simulink model "Paper_Simulation_final"  (R2020a)
settings: Solver=ode15s  StartTime=0.0  StopTime=1  MaxStep=0.000002  MinStep=2e-12  RelTol=1e-3
model workspace (MAT data in the model file):
  Wo = 1
  wfinal = Simulink.Parameter
  wfinal.DataType = 'auto'
  wfinal.Dimensions = [0 0]
values from neighbouring files (symbols this model uses):
  a = sqrt(2)*sigma    [tune.m]
  A = conv(A,[1 .5 1])    [tune.m]
  ades = 2*zeta    [tune.m]
  B = conv(B,[-1.5 1])    [tune.m]
  beta = beta/fact    (= 0.5)    [tune.m]
  d = [0*(1:Td/h) 1]    [tune.m]
  d1 = [0*(1:round(Tdhat/h)) 1]    [tune.m]
  h = Tmax/Npts    [tune.m]
  K = K/fact    [tune.m]
  K0 = 1/Kp0    [tune.m]
  K_hat = TThat*ppp(2)/stepsize    [tune.m]
  kfinal = 1/Kw    [tune.m]
  Kmult = 1*Kmult    [tune.m]
  load_s = -0.000    (= 0)    [tune.m]
  phi_c = -1.25; end    [tune.m]
  SetPoint = 1    [tune.m]
  Sn = Snset*st    (= 0)    [tune.m]
  st = 0.1    [tune.m]
  stepsize = 1/Tmax    [tune.m]
  T_l = 0    [tune.m]
  Td = max(h*round(Td/h),h)    [tune.m]
  Tf = Tf*fact    [tune.m]
  Tmax = Tmax_n    [tune.m]
  Tmax_c = Tmax_c+T_l    [tune.m]
  Ts = max((2*Tmhat-Tdhat),ty2)    [tune.m]
  Tsw = max(10*Tmhat,5/(beta*wbar))    [tune.m]
  TswK = Tsw/2    [tune.m]
  TThat = -0.5*ppp(2)/ppp(1)    [tune.m]
  wbar = wbar_n    [tune.m]
  wfinal = wbar_n    [tune.m]
undefined symbols (not defined in the file or in its folder): fdesignblkfcn, gcbh, tstop
libraries: simulink x3, simulink_extras x3, powerlib_meascontrol x2
settings Model: Creator=Ayush Agrawal  LastModifiedBy=Ayush Agrawal
settings SolverCC: InitialStep=2e-6  ZeroCrossAlgorithm=Adaptive
settings DebuggingCC: AlgebraicLoopMsg=none

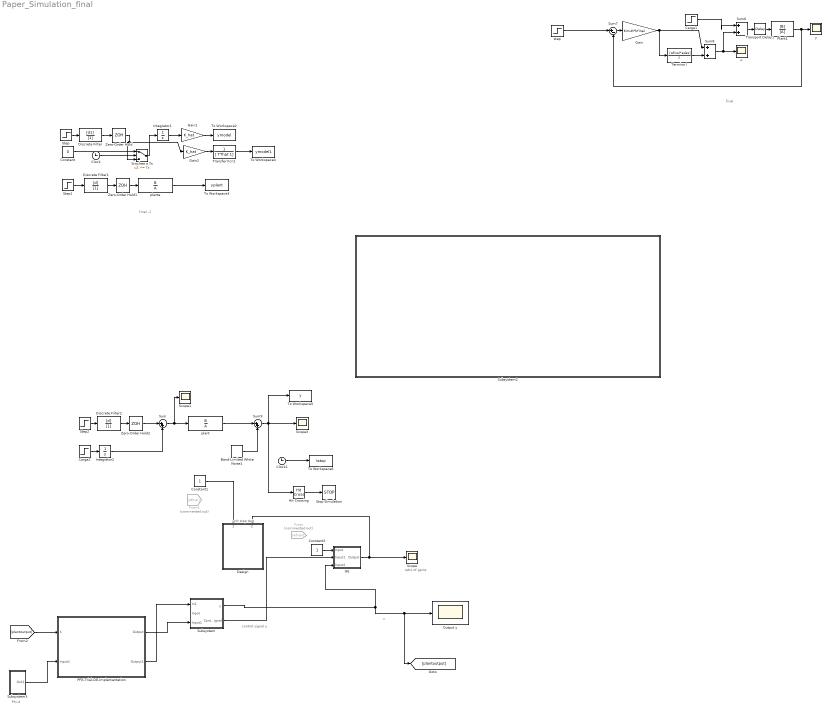
== system Paper_Simulation_final ==
  note: ratio of gains
  note: x
  note: Phi-d
  note: control signal
      |         u
  note: final -1
  note: final
  note: unit step test
  Band-Limited White Noise1 : simulink/Sources/Band-Limited White Noise  Cov=[Sn]  Ts=h  seed=[23341]
  Carga1 : Step  Time=0  After=load  SampleTime=0
  Carga2 : Step  Time=T_l  After=load_s  SampleTime=0
  Clock : Clock
  Clock1 : Clock
  Constant : Constant  Value=0
  Constant1 : Constant
  Constant2 : Constant
  Design : Subsystem  mask{a=1.5}
  Discrete Filter : DiscreteFilter  Numerator=[d1]  Denominator=[1]  SampleTime=h
  Discrete Filter1 : DiscreteFilter  Numerator=[d]  Denominator=[1]  SampleTime=h
  Discrete Filter2 : DiscreteFilter  Numerator=[d]  Denominator=[1]  SampleTime=h
  From : From  Commented=on  GotoTag=wfinal
  From1 : From  Commented=on  GotoTag=wfinal
  GE : Subsystem  mask{winitial=10}
  Gain : Gain  Gain=Kmult*kfinal  SaturateOnIntegerOverflow=on  OutDataTypeStr=Inherit: Same as input  ParamDataTypeStr=Inherit: Same as input
  Gain1 : Gain  Gain=K_hat  SaturateOnIntegerOverflow=on  OutDataTypeStr=Inherit: Same as input  ParamDataTypeStr=Inherit: Same as input
  Gain2 : Gain  Gain=K_hat  SaturateOnIntegerOverflow=on  OutDataTypeStr=Inherit: Same as input  ParamDataTypeStr=Inherit: Same as input
  Hit Crossing : HitCross  HitCrossingOffset=Y2  HitCrossingDirection=rising
  Integrator1 : Integrator
  Integrator2 : Integrator
  Output y : Scope
  PFE-Trial-DE-Implementation : Subsystem  mask{winitial=10}
  Plant1 : TransferFcn  Numerator=[B]  Denominator=[A]
  Scope : Scope
  Scope1 : Scope
  Scope3 : Scope
  Siwchea a Ts : Switch  Threshold=Ts  SaturateOnIntegerOverflow=on
  Step : Step  Time=0  After=stepsize  SampleTime=h
  Step1 : Step  Time=0  After=stepsize  SampleTime=h
  Step2 : Step  Time=0  After=stepsize  SampleTime=h
  Stop Simulation : Stop
  Subsystem : Subsystem  mask{Ti=1, r=0.25}
  Subsystem2 : Subsystem
  Subsystem3 : Subsystem  mask{Phid=10}
      mask prompts: Phid "Phi-d"
  Sum{,6,8..9} (4 alike) : Sum  Inputs=|++  InputSameDT=on  SaturateOnIntegerOverflow=on  OutDataTypeStr=Inherit: Same as first input
  Sum7 : Sum  Inputs=|+-  InputSameDT=on  SaturateOnIntegerOverflow=on  OutDataTypeStr=Inherit: Same as first input
  Termino I : TransferFcn  Numerator=[wfinal*ades]  Denominator=[1 0]
  To Workspace2 : ToWorkspace  VariableName=ymodel  SampleTime=h
  To Workspace3 : ToWorkspace  VariableName=yplant  SampleTime=h
  To Workspace4 : ToWorkspace  VariableName=ymodel1  SampleTime=h
  To Workspace5 : ToWorkspace  VariableName=y  SampleTime=h
  To Workspace6 : ToWorkspace  VariableName=tstop  SampleTime=h
      settings: MaxDataPoints=1
  Transfer Fcn1 : TransferFcn  Denominator=[ TThat 1]
  Transport Delay1 : TransportDelay  DelayTime=Td  BufferSize=16384
  Zero-Order Hold : ZeroOrderHold  SampleTime=h
  Zero-Order Hold1 : ZeroOrderHold  SampleTime=h
  Zero-Order Hold2 : ZeroOrderHold  SampleTime=h
  plant : TransferFcn  Numerator=B  Denominator=A
  planta : TransferFcn  Numerator=B  Denominator=A
  step : Step  Time=0  After=SetPoint  SampleTime=0
  u : Scope
  y : Scope
  wires:
  Subsystem/1(y) -> GE/3(Input2), [plantoutput], Output y/1
  GE/1(Output) -> Scope/1, Design/2(Plant Gain Amplitude)
  Subsystem3/1(Out1) -> PFE-Trial-DE-Implementation/2(Input1)
  [plantoutput] -> PFE-Trial-DE-Implementation/1(X)
  Subsystem/2(Control SIgnal) -> GE/2(Input1)
  Constant1/1 -> Design/1(PFE O/P frequency)
  Constant2/1 -> GE/1(Input)
  PFE-Trial-DE-Implementation/1(Output) -> Subsystem/3(Input1)
  PFE-Trial-DE-Implementation/2(Output1) -> Subsystem/1(In1)
  Transfer Fcn1/1 -> To Workspace4/1
  Discrete Filter1/1 -> Zero-Order Hold1/1
  Gain2/1 -> Transfer Fcn1/1
  Integrator1/1 -> Gain1/1
  Step1/1 -> Discrete Filter1/1
  Siwchea a Ts/1 -> Integrator1/1
  Constant/1 -> Siwchea a Ts/1
  Step/1 -> Discrete Filter/1
  Discrete Filter/1 -> Zero-Order Hold/1
  Zero-Order Hold/1 -> Siwchea a Ts/3, Gain2/1
  planta/1 -> To Workspace3/1
  Gain1/1 -> To Workspace2/1
  Clock/1 -> Siwchea a Ts/2
  Zero-Order Hold1/1 -> planta/1
  Plant1/1 -> Sum7/2, y/1
  Sum7/1 -> Gain/1
  Sum8/1 -> Sum6/2, u/1
  Carga1/1 -> Sum6/1
  step/1 -> Sum7/1
  Gain/1 -> Sum8/1, Termino I/1
  Termino I/1 -> Sum8/2
  Transport Delay1/1 -> Plant1/1
  Sum6/1 -> Transport Delay1/1
  Discrete Filter2/1 -> Zero-Order Hold2/1
  Carga2/1 -> Integrator2/1
  Step2/1 -> Discrete Filter2/1
  Hit Crossing/1 -> Stop Simulation/1
  Band-Limited White Noise1/1 -> Sum9/2
  Zero-Order Hold2/1 -> Sum/1
  Integrator2/1 -> Sum/2
  Clock1/1 -> To Workspace6/1
  Sum9/1 -> Scope3/1, To Workspace5/1, Hit Crossing/1
  plant/1 -> Sum9/1
  Sum/1 -> plant/1, Scope1/1

== system Paper_Simulation_final/Design ==
  PFE O/P frequency : Inport
  Plant Gain Amplitude : Inport  Port=2
  Goto1 : Goto  Commented=on  GotoTag=Ti  TagVisibility=global
  Scope : Scope
  Scope1 : Scope
  Subsystem : Subsystem
  tag scope: K=global
  wires:
  PFE O/P frequency/1 -> Subsystem/1(PFE O/P freq)
  Plant Gain Amplitude/1 -> Subsystem/2(Input)
  Subsystem/1(K) -> Scope/1, [K]
  Subsystem/2(Ti) -> Scope1/1, Goto1/1

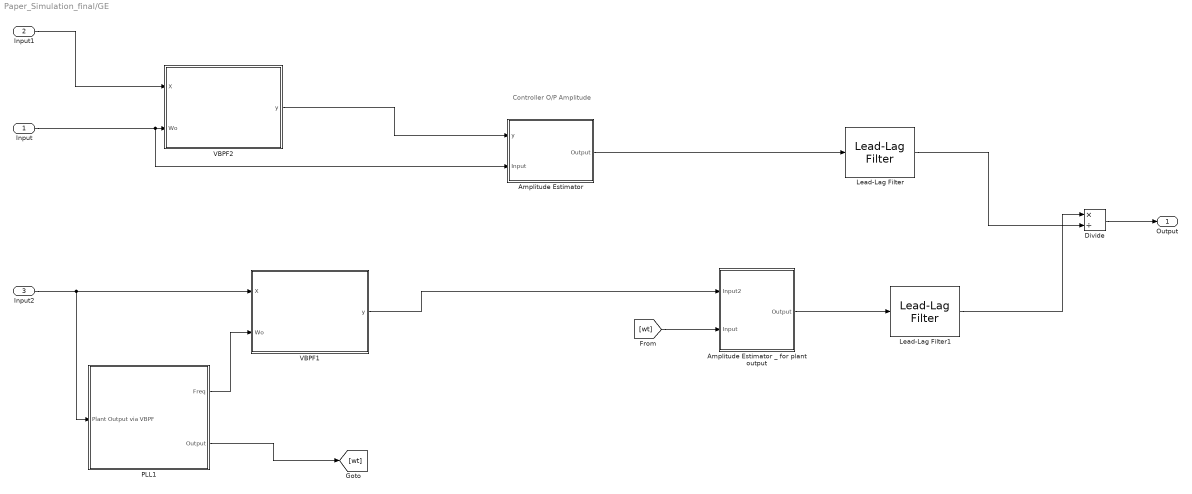
== system Paper_Simulation_final/GE ==
  note: Controller O/P Amplitude
  Input : Inport
  Input1 : Inport  Port=2
  Input2 : Inport  Port=3
  Amplitude Estimator : Subsystem
  Amplitude Estimator _ for plant output : Subsystem
  Divide : Product  Inputs=*/
  Lead-Lag Filter : powerlib_meascontrol/Filters/Lead-Lag Filter  T1=0  T2=10/winitial  Vdc_Init=0  Ts=0.1
      settings: SourceProductBaseCode=PS
  Lead-Lag Filter1 : powerlib_meascontrol/Filters/Lead-Lag Filter  T1=0  T2=10/winitial  Vdc_Init=0  Ts=0
      settings: SourceProductBaseCode=PS
  PLL1 : Subsystem
  VBPF1 : Subsystem
  VBPF2 : Subsystem
  Output : Outport
  wires:
  Input1/1 -> VBPF2/1(X)
  Input2/1 -> PLL1/1(Plant Output via VBPF), VBPF1/1(X)
  Amplitude Estimator _ for plant output/1(Output) -> Lead-Lag Filter1/1
  Divide/1 -> Output/1
  Lead-Lag Filter1/1 -> Divide/1
  Lead-Lag Filter/1 -> Divide/2
  PLL1/1(Freq) -> VBPF1/2(Wo)
  PLL1/2(Output) -> [wt]
  Input/1 -> Amplitude Estimator/2(Input), VBPF2/2(Wo)
  VBPF1/1(y) -> Amplitude Estimator _ for plant output/1(Input2)
  VBPF2/1(y) -> Amplitude Estimator/1(y)
  [wt] -> Amplitude Estimator _ for plant output/2(Input)
  Amplitude Estimator/1(Output) -> Lead-Lag Filter/1

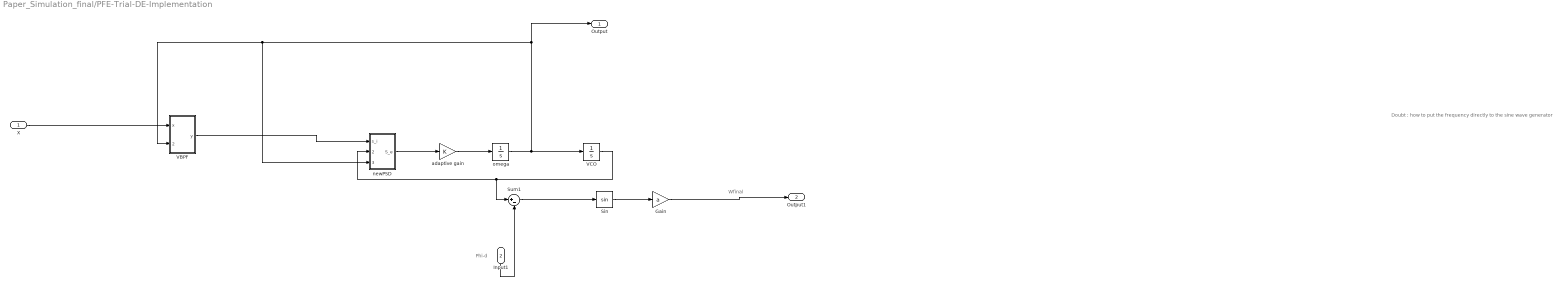
== system Paper_Simulation_final/PFE-Trial-DE-Implementation ==
  note: Doubt : how to put the frequency directly to the sine wave generator
  note: Wfinal
  note: Phi-d
  X : Inport
  Input1 : Inport  Port=2
  "   adaptive gain" : Gain  Gain=K  SaturateOnIntegerOverflow=on  OutDataTypeStr=Inherit: Same as input  ParamDataTypeStr=Inherit: Same as input
  Gain : Gain  Gain=a
  Sin : Trigonometry
  Sum1 : Sum  Inputs=|+-
  VBPF : Subsystem
  "VCO " : Integrator  InitialCondition=-pi  LowerSaturationLimit=0.5
  newPSD : Subsystem
  omega : Integrator  InitialCondition=wbar  LowerSaturationLimit=wbar/3
  Output : Outport
  Output1 : Outport  Port=2
  wires:
  Input1/1 -> Sum1/2
  X/1 -> VBPF/1(x)
  Sum1/1 -> Sin/1
  Sin/1 -> Gain/1
  Gain/1 -> Output1/1
  ? -> ?
  VBPF/1(y) -> newPSD/1(s_i)
  newPSD/1(S_e) -> "   adaptive gain"/1
  "   adaptive gain"/1 -> omega/1
  omega/1 -> Output/1, VBPF/2(omega_0), newPSD/3(omega_o), "VCO "/1
  "VCO "/1 -> newPSD/2(phi_o), Sum1/1

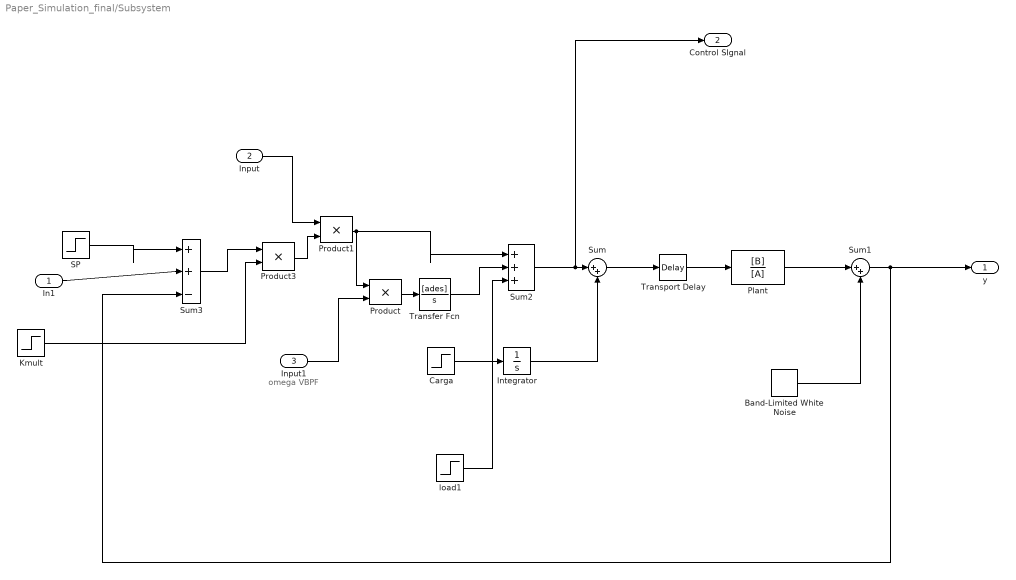
== system Paper_Simulation_final/Subsystem ==
  note: omega VBPF
  In1 : Inport
  Input : Inport  Port=2
  Input1 : Inport  Port=3
  Band-Limited White Noise : simulink/Sources/Band-Limited White Noise  Cov=[Sn]  Ts=st  seed=[23341]
  Carga : Step  Time=T_l  After=load_s  SampleTime=0
  Integrator : Integrator
  Kmult : Step  Time=tstop  After=Kmult  SampleTime=0
  Plant : TransferFcn  Numerator=[B]  Denominator=[A]
  Product : Product  InputSameDT=on  SaturateOnIntegerOverflow=on  OutDataTypeStr=Inherit: Same as first input
  Product1 : Product  InputSameDT=on  SaturateOnIntegerOverflow=on  OutDataTypeStr=Inherit: Same as first input
  Product3 : Product  InputSameDT=on  SaturateOnIntegerOverflow=on  OutDataTypeStr=Inherit: Same as first input
  SP : Step  Time=Tmax_c/2  Before=SetPoint  After=SetPoint  SampleTime=0
  Sum : Sum  Inputs=|++
  Sum1 : Sum  Inputs=|++  InputSameDT=on  SaturateOnIntegerOverflow=on  OutDataTypeStr=Inherit: Same as first input
  Sum2 : Sum  Inputs=|+++
  Sum3 : Sum  Inputs=|++-  InputSameDT=on  SaturateOnIntegerOverflow=on  OutDataTypeStr=Inherit: Same as first input
  Transfer Fcn : TransferFcn  Numerator=[ades]  Denominator=[1 0]
  Transport Delay : TransportDelay  DelayTime=Td  BufferSize=65536
  load1 : Step  Time=Tmax  Before=stepsize  After=stepsize  SampleTime=0
  y : Outport
  Control SIgnal : Outport  Port=2
  wires:
  Plant/1 -> Sum1/1
  Band-Limited White Noise/1 -> Sum1/2
  Transport Delay/1 -> Plant/1
  Sum/1 -> Transport Delay/1
  Carga/1 -> Integrator/1
  Integrator/1 -> Sum/2
  Sum2/1 -> Control SIgnal/1, Sum/1
  Transfer Fcn/1 -> Sum2/2
  load1/1 -> Sum2/3
  In1/1 -> Sum3/2
  SP/1 -> Sum3/1
  Sum3/1 -> Product3/1
  Kmult/1 -> Product3/2
  Sum1/1 -> Sum3/3, y/1
  Product3/1 -> Product1/2
  Input/1 -> Product1/1
  Product/1 -> Transfer Fcn/1
  Product1/1 -> Product/1, Sum2/1
  Input1/1 -> Product/2

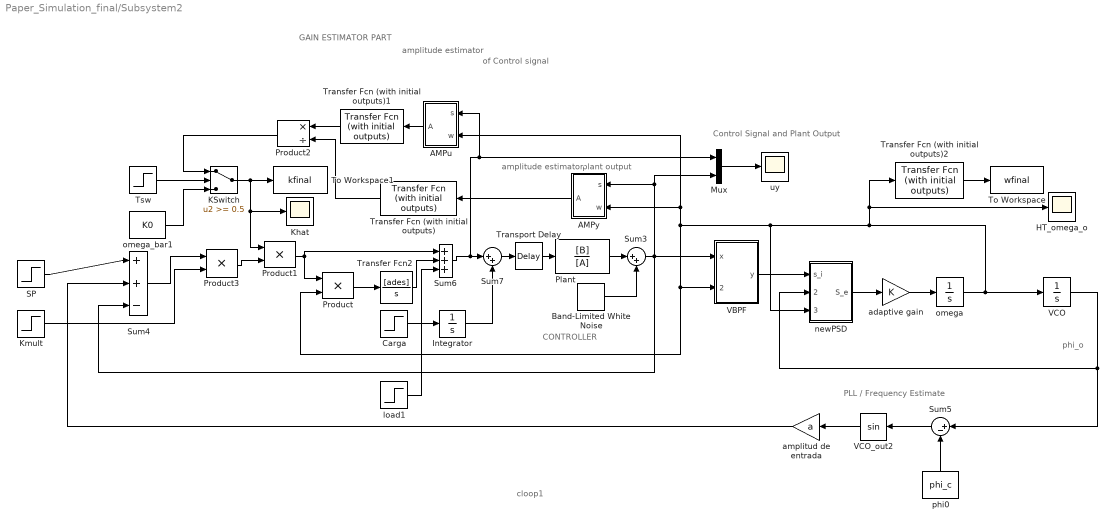
== system Paper_Simulation_final/Subsystem2 ==
  note: plant output
  note: CONTROLLER
  note: amplitude estimator
  note: cloop1
  note: Control Signal and Plant Output
  note: of Control signal
  note: PLL / Frequency Estimate
  note: GAIN ESTIMATOR PART
  note: phi_o
  note: amplitude estimator
  "   adaptive gain" : Gain  Gain=K  SaturateOnIntegerOverflow=on  OutDataTypeStr=Inherit: Same as input  ParamDataTypeStr=Inherit: Same as input
  "   amplitud de entrada" : Gain  Gain=a  SaturateOnIntegerOverflow=on  OutDataTypeStr=Inherit: Same as input  ParamDataTypeStr=Inherit: Same as input
  AMPu : Subsystem
  AMPy : Subsystem
  Band-Limited White Noise : simulink/Sources/Band-Limited White Noise  Cov=[Sn]  Ts=st  seed=[23341]
  Carga : Step  Time=T_l  After=load_s  SampleTime=0
  HT_omega_o : Scope
  Integrator : Integrator
  KSwitch : Switch  Threshold=0.5  ZeroCross=off  SaturateOnIntegerOverflow=on  InputSameDT=on
  Khat : Scope
  Kmult : Step  Time=tstop  After=Kmult  SampleTime=0
  Mux : Mux  Inputs=2
  Plant : TransferFcn  Numerator=[B]  Denominator=[A]
  Product : Product  InputSameDT=on  SaturateOnIntegerOverflow=on  OutDataTypeStr=Inherit: Same as first input
  Product1 : Product  InputSameDT=on  SaturateOnIntegerOverflow=on  OutDataTypeStr=Inherit: Same as first input
  Product2 : Product  Inputs=*/  InputSameDT=on  SaturateOnIntegerOverflow=on  OutDataTypeStr=Inherit: Same as first input
  Product3 : Product  InputSameDT=on  SaturateOnIntegerOverflow=on  OutDataTypeStr=Inherit: Same as first input
  SP : Step  Time=Tmax_c/2  Before=SetPoint  After=SetPoint  SampleTime=0
  Sum3 : Sum  Inputs=|++  InputSameDT=on  SaturateOnIntegerOverflow=on  OutDataTypeStr=Inherit: Same as first input
  Sum4 : Sum  Inputs=|++-  InputSameDT=on  SaturateOnIntegerOverflow=on  OutDataTypeStr=Inherit: Same as first input
  Sum5 : Sum  Inputs=|+-  InputSameDT=on  SaturateOnIntegerOverflow=on  OutDataTypeStr=Inherit: Same as first input
  Sum6 : Sum  Inputs=|+++  InputSameDT=on  SaturateOnIntegerOverflow=on  OutDataTypeStr=Inherit: Same as first input
  Sum7 : Sum  Inputs=|++  InputSameDT=on  SaturateOnIntegerOverflow=on  OutDataTypeStr=Inherit: Same as first input
  To Workspace : ToWorkspace  VariableName=wfinal  SampleTime=-1
      settings: MaxDataPoints=1
  To Workspace1 : ToWorkspace  VariableName=kfinal
      settings: MaxDataPoints=1
  Transfer Fcn (with initial outputs) : simulink_extras/Additional Linear/Transfer Fcn (with initial outputs)  N=[1]  D="[Tf  1]"  Y0=a  U0=a
  Transfer Fcn (with initial outputs)1 : simulink_extras/Additional Linear/Transfer Fcn (with initial outputs)  N=[1]  D="[Tf  1]"  Y0=K0*a  U0=K0*a
  Transfer Fcn (with initial outputs)2 : simulink_extras/Additional Linear/Transfer Fcn (with initial outputs)  N=[1]  D="[Tf  1]"  Y0=wbar  U0=wbar
  Transfer Fcn2 : TransferFcn  Numerator=[ades]  Denominator=[1 0]
  Transport Delay : TransportDelay  DelayTime=Td  BufferSize=65536
  Tsw : Step  Time=TswK+tstop  SampleTime=0
  VBPF : Subsystem
  "VCO " : Integrator  InitialCondition=-pi  LowerSaturationLimit=0.5
  VCO_out2 : Trigonometry
  load1 : Step  Time=Tmax  Before=stepsize  After=stepsize  SampleTime=0
  newPSD : Subsystem
  omega : Integrator  InitialCondition=wbar  LowerSaturationLimit=wbar/3
  omega_bar1 : Constant  Value=K0
  phi0 : Constant  Value=phi_c
  uy : Scope
  wires:
  Tsw/1 -> KSwitch/2
  "   amplitud de entrada"/1 -> Sum4/2
  Kmult/1 -> Product3/2
  Integrator/1 -> Sum7/2
  VCO_out2/1 -> "   amplitud de entrada"/1
  Product3/1 -> Product1/2
  AMPu/1(A) -> Transfer Fcn (with initial outputs)1/1
  omega/1 -> Transfer Fcn (with initial outputs)2/1, HT_omega_o/1, VBPF/2(omega_0), Product/2, AMPu/2(w), AMPy/2(w), newPSD/3(omega_o), "VCO "/1
  Band-Limited White Noise/1 -> Sum3/2
  Sum7/1 -> Transport Delay/1
  phi0/1 -> Sum5/2
  Mux/1 -> uy/1
  Transfer Fcn (with initial outputs)2/1 -> To Workspace/1
  Carga/1 -> Integrator/1
  Product1/1 -> Product/1, Sum6/1
  Transport Delay/1 -> Plant/1
  SP/1 -> Sum4/1
  Transfer Fcn (with initial outputs)1/1 -> Product2/1
  Sum3/1 -> VBPF/1(x), AMPy/1(s), Mux/2, Sum4/3
  KSwitch/1 -> Product1/1, Khat/1, To Workspace1/1
  newPSD/1(S_e) -> "   adaptive gain"/1
  Product2/1 -> KSwitch/1
  AMPy/1(A) -> Transfer Fcn (with initial outputs)/1
  Transfer Fcn2/1 -> Sum6/2
  "VCO "/1 -> Sum5/1, newPSD/2(phi_o)
  omega_bar1/1 -> KSwitch/3
  Sum5/1 -> VCO_out2/1
  load1/1 -> Sum6/3
  "   adaptive gain"/1 -> omega/1
  Transfer Fcn (with initial outputs)/1 -> Product2/2
  Sum6/1 -> AMPu/1(s), Mux/1, Sum7/1
  Sum4/1 -> Product3/1
  Plant/1 -> Sum3/1
  Product/1 -> Transfer Fcn2/1
  VBPF/1(y) -> newPSD/1(s_i)

== system Paper_Simulation_final/Subsystem3 ==
  Constant1 : Constant
  Out1 : Outport
  wires:
  Constant1/1 -> Out1/1

== system Paper_Simulation_final/Design/Subsystem ==
  note: Used for calculating P Gain for our controller
  note: Integral Time
  note: Plant Gain
  PFE O/P freq : Inport
  Input : Inport  Port=2
  Subsystem : Subsystem
  Subsystem1 : Subsystem
  K : Outport
  Ti : Outport  Port=2
  wires:
  Input/1 -> Subsystem/1(Plant Gain)
  Subsystem/1(K) -> K/1
  PFE O/P freq/1 -> Subsystem1/1(PFE O/P freq)
  Subsystem1/1(Ti) -> Ti/1

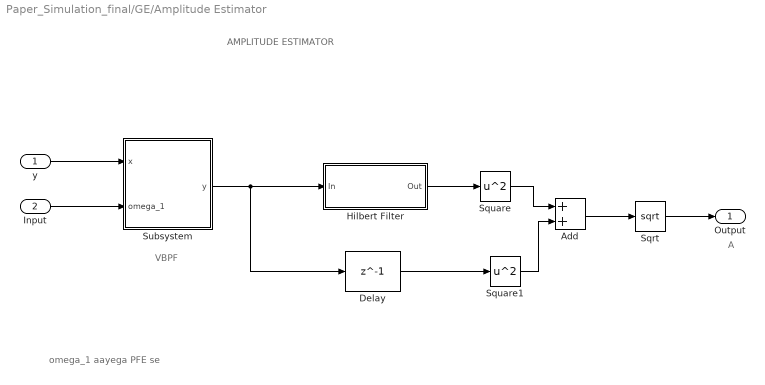
== system Paper_Simulation_final/GE/Amplitude Estimator ==
  note: omega_1 aayega PFE se
  note: A
  note: AMPLITUDE ESTIMATOR
  note: VBPF
  y : Inport
  Input : Inport  Port=2
  Add : Sum
  Delay : Delay  DelayLength=1  InitialCondition=0  UseCircularBuffer=on
  Hilbert Filter : Subsystem  DialogController=fdesignblkfcn  InitFcn=fdesignblkfcn(gcbh, {'InitFcn'});  mask(Hilbert Filter){}
      mask help: Design a Hilbert filter
      settings: CopyFcn=fdesignblkfcn(gcbh, {'CopyFcn'});
      mask Help: helpview(mapfilelocation('dsp'), 'dsphilbertfilter');
      mask Display: disp('Hilbert')
  Sqrt : Sqrt  SaturateOnIntegerOverflow=on
  Square : Math  Operator=square  SaturateOnIntegerOverflow=on
  Square1 : Math  Operator=square  SaturateOnIntegerOverflow=on
  Subsystem : Subsystem
  Output : Outport
  wires:
  Input/1 -> Subsystem/2(omega_1)
  y/1 -> Subsystem/1(x)
  Subsystem/1(y) -> Delay/1, Hilbert Filter/1(In)
  Hilbert Filter/1(Out) -> Square/1
  Delay/1 -> Square1/1
  Square/1 -> Add/1
  Square1/1 -> Add/2
  Add/1 -> Sqrt/1
  Sqrt/1 -> Output/1

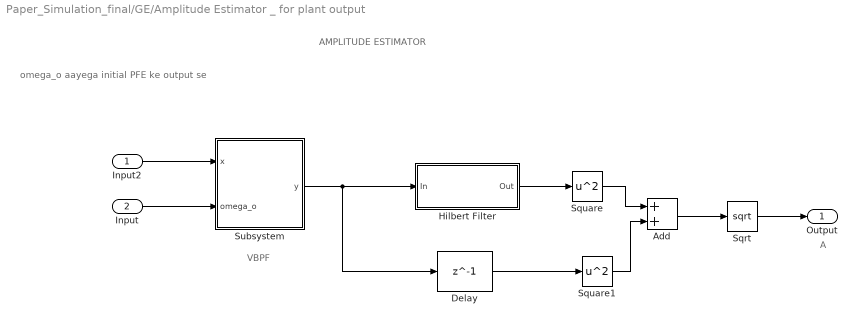
== system Paper_Simulation_final/GE/Amplitude Estimator _ for plant output ==
  note: omega_o aayega initial PFE ke output se
  note: A
  note: AMPLITUDE ESTIMATOR
  note: VBPF
  Input2 : Inport
  Input : Inport  Port=2
  Add : Sum
  Delay : Delay  DelayLength=1  InitialCondition=0  UseCircularBuffer=on
  Hilbert Filter : Subsystem  DialogController=fdesignblkfcn  InitFcn=fdesignblkfcn(gcbh, {'InitFcn'});  mask(Hilbert Filter){}
      mask help: Design a Hilbert filter
      settings: CopyFcn=fdesignblkfcn(gcbh, {'CopyFcn'});
      mask Help: helpview(mapfilelocation('dsp'), 'dsphilbertfilter');
      mask Display: disp('Hilbert')
  Sqrt : Sqrt  SaturateOnIntegerOverflow=on
  Square : Math  Operator=square  SaturateOnIntegerOverflow=on
  Square1 : Math  Operator=square  SaturateOnIntegerOverflow=on
  Subsystem : Subsystem
  Output : Outport
  wires:
  Input/1 -> Subsystem/2(omega_o)
  Input2/1 -> Subsystem/1(x)
  Subsystem/1(y) -> Delay/1, Hilbert Filter/1(In)
  Hilbert Filter/1(Out) -> Square/1
  Delay/1 -> Square1/1
  Square/1 -> Add/1
  Square1/1 -> Add/2
  Add/1 -> Sqrt/1
  Sqrt/1 -> Output/1

== system Paper_Simulation_final/GE/PLL1 ==
  note: present phase
  Plant Output via VBPF : Inport
  Cos : Trigonometry  Operator=cos
  Integrator1 : Integrator
  PSD : Subsystem
  Transfer Fcn : TransferFcn  Numerator=[1 1]  Denominator=[1 1 0]
  Freq : Outport
  Output : Outport  Port=2
  wires:
  Cos/1 -> PSD/2(Input)
  PSD/1(Out1) -> Transfer Fcn/1
  Plant Output via VBPF/1 -> PSD/1(In1)
  Integrator1/1 -> Output/1, Cos/1
  Transfer Fcn/1 -> Freq/1, Integrator1/1

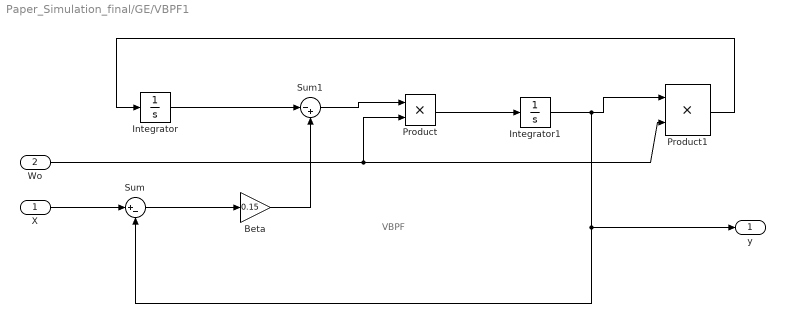
== system Paper_Simulation_final/GE/VBPF1 ==
  note: VBPF
  X : Inport
  Wo : Inport  Port=2
  Beta : Gain  Gain=0.15
  Integrator : Integrator
  Integrator1 : Integrator
  Product : Product
  Product1 : Product
  Sum : Sum  Inputs=|+-
  Sum1 : Sum  Inputs=|-+
  y : Outport
  wires:
  X/1 -> Sum/1
  Sum/1 -> Beta/1
  Integrator/1 -> Sum1/1
  Beta/1 -> Sum1/2
  Sum1/1 -> Product/1
  Wo/1 -> Product1/2, Product/2
  Product/1 -> Integrator1/1
  Integrator1/1 -> Product1/1, Sum/2, y/1
  Product1/1 -> Integrator/1

== system Paper_Simulation_final/GE/VBPF2 ==
  note: VBPF
  X : Inport
  Wo : Inport  Port=2
  Beta : Gain  Gain=1.5
  Integrator : Integrator
  Integrator1 : Integrator  LimitOutput=on  UpperSaturationLimit=10  LowerSaturationLimit=-10
  Product : Product
  Product1 : Product
  Sum : Sum  Inputs=|+-
  Sum1 : Sum  Inputs=|-+
  y : Outport
  wires:
  X/1 -> Sum/1
  Sum/1 -> Beta/1
  Integrator/1 -> Sum1/1
  Beta/1 -> Sum1/2
  Sum1/1 -> Product/1
  Wo/1 -> Product1/2, Product/2
  Product/1 -> Integrator1/1
  Integrator1/1 -> Product1/1, Sum/2, y/1
  Product1/1 -> Integrator/1

== system Paper_Simulation_final/PFE-Trial-DE-Implementation/VBPF ==
  note: Variable BPF
  x : Inport
  omega_0 : Inport  Port=2
  Integrator : Integrator
  Integrator1 : Integrator
  Product : Product  InputSameDT=on  SaturateOnIntegerOverflow=on  OutDataTypeStr=Inherit: Same as first input
  Product1 : Product  InputSameDT=on  SaturateOnIntegerOverflow=on  OutDataTypeStr=Inherit: Same as first input
  Sum : Sum  Inputs=|-+  InputSameDT=on  SaturateOnIntegerOverflow=on  OutDataTypeStr=Inherit: Same as first input
  Sum1 : Sum  Inputs=|+-  InputSameDT=on  SaturateOnIntegerOverflow=on  OutDataTypeStr=Inherit: Same as first input
  beta : Gain  Gain=beta  SaturateOnIntegerOverflow=on  OutDataTypeStr=Inherit: Same as input  ParamDataTypeStr=Inherit: Same as input
  y : Outport
  wires:
  beta/1 -> Sum/2
  Sum1/1 -> beta/1
  Product/1 -> Integrator/1
  Integrator1/1 -> Sum/1
  Product1/1 -> Integrator1/1
  Integrator/1 -> Sum1/2, y/1, Product1/1
  omega_0/1 -> Product/2, Product1/2
  Sum/1 -> Product/1
  x/1 -> Sum1/1

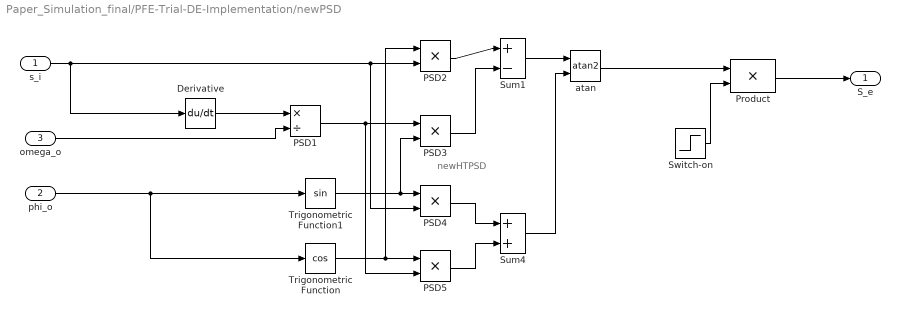
== system Paper_Simulation_final/PFE-Trial-DE-Implementation/newPSD ==
  note: newHTPSD
  s_i : Inport
  phi_o : Inport  Port=2
  omega_o : Inport  Port=3
  Derivative : Derivative
  PSD1 : Product  Inputs=*/  InputSameDT=on  SaturateOnIntegerOverflow=on  OutDataTypeStr=Inherit: Same as first input
  PSD{2..5} (4 alike) : Product  Inputs=**  InputSameDT=on  SaturateOnIntegerOverflow=on  OutDataTypeStr=Inherit: Same as first input
  Product : Product  InputSameDT=on  SaturateOnIntegerOverflow=on  OutDataTypeStr=Inherit: Same as first input
  Sum1 : Sum  Inputs=|+-  InputSameDT=on  SaturateOnIntegerOverflow=on  OutDataTypeStr=Inherit: Same as first input
  Sum4 : Sum  InputSameDT=on  SaturateOnIntegerOverflow=on  OutDataTypeStr=Inherit: Same as first input
  Switch-on : Step  Time=Tsw+tstop  SampleTime=0
  Trigonometric Function : Trigonometry  Operator=cos
  Trigonometric Function1 : Trigonometry
  atan : Trigonometry  Operator=atan2
  S_e : Outport
  wires:
  omega_o/1 -> PSD1/2
  PSD1/1 -> PSD5/2, PSD3/1
  Derivative/1 -> PSD1/1
  PSD2/1 -> Sum1/1
  PSD3/1 -> Sum1/2
  Sum1/1 -> atan/1
  PSD4/1 -> Sum4/1
  PSD5/1 -> Sum4/2
  Sum4/1 -> atan/2
  s_i/1 -> PSD4/2, PSD2/2, Derivative/1
  Trigonometric Function/1 -> PSD2/1, PSD5/1
  Trigonometric Function1/1 -> PSD3/2, PSD4/1
  phi_o/1 -> Trigonometric Function1/1, Trigonometric Function/1
  atan/1 -> Product/1
  Product/1 -> S_e/1
  Switch-on/1 -> Product/2

== system Paper_Simulation_final/Subsystem2/AMPu ==
  s : Inport
  w : Inport  Port=2
  Derivative : Derivative
  Math Function : Math  Operator=square  SignedPower=on  SaturateOnIntegerOverflow=on
  Math Function1 : Math  Operator=square  SignedPower=on  SaturateOnIntegerOverflow=on
  Math Function2 : Math  Operator=sqrt  SignedPower=on  SaturateOnIntegerOverflow=on
  Product : Product  Inputs=*/  SaturateOnIntegerOverflow=on  OutDataTypeStr=Inherit: Same as first input
  Sum2 : Sum  InputSameDT=on  SaturateOnIntegerOverflow=on  OutDataTypeStr=Inherit: Same as first input
  VBPF : Subsystem
  A : Outport
  wires:
  Product/1 -> Math Function1/1
  Sum2/1 -> Math Function2/1
  Math Function2/1 -> A/1
  Math Function/1 -> Sum2/1
  Math Function1/1 -> Sum2/2
  s/1 -> VBPF/1(x)
  w/1 -> Product/2, VBPF/2(omega_0)
  VBPF/1(y) -> Math Function/1, Derivative/1
  Derivative/1 -> Product/1

== system Paper_Simulation_final/Subsystem2/AMPy ==
  s : Inport
  w : Inport  Port=2
  Derivative : Derivative
  Math Function : Math  Operator=square  SignedPower=on  SaturateOnIntegerOverflow=on
  Math Function1 : Math  Operator=square  SignedPower=on  SaturateOnIntegerOverflow=on
  Math Function2 : Math  Operator=sqrt  SignedPower=on  SaturateOnIntegerOverflow=on
  Product : Product  Inputs=*/  SaturateOnIntegerOverflow=on  OutDataTypeStr=Inherit: Same as first input
  Sum2 : Sum  InputSameDT=on  SaturateOnIntegerOverflow=on  OutDataTypeStr=Inherit: Same as first input
  VBPF : Subsystem
  A : Outport
  wires:
  w/1 -> VBPF/2(omega_0), Product/2
  s/1 -> VBPF/1(x)
  Math Function1/1 -> Sum2/2
  Math Function/1 -> Sum2/1
  Math Function2/1 -> A/1
  Sum2/1 -> Math Function2/1
  Product/1 -> Math Function1/1
  VBPF/1(y) -> Math Function/1, Derivative/1
  Derivative/1 -> Product/1

== system Paper_Simulation_final/Subsystem2/VBPF ==
  note: Variable BPF
  x : Inport
  omega_0 : Inport  Port=2
  Integrator : Integrator
  Integrator1 : Integrator
  Product : Product  InputSameDT=on  SaturateOnIntegerOverflow=on  OutDataTypeStr=Inherit: Same as first input
  Product1 : Product  InputSameDT=on  SaturateOnIntegerOverflow=on  OutDataTypeStr=Inherit: Same as first input
  Sum : Sum  Inputs=|-+  InputSameDT=on  SaturateOnIntegerOverflow=on  OutDataTypeStr=Inherit: Same as first input
  Sum1 : Sum  Inputs=|+-  InputSameDT=on  SaturateOnIntegerOverflow=on  OutDataTypeStr=Inherit: Same as first input
  beta : Gain  Gain=beta  SaturateOnIntegerOverflow=on  OutDataTypeStr=Inherit: Same as input  ParamDataTypeStr=Inherit: Same as input
  y : Outport
  wires:
  beta/1 -> Sum/2
  Sum1/1 -> beta/1
  Product/1 -> Integrator/1
  Integrator1/1 -> Sum/1
  Product1/1 -> Integrator1/1
  Integrator/1 -> Sum1/2, y/1, Product1/1
  omega_0/1 -> Product/2, Product1/2
  Sum/1 -> Product/1
  x/1 -> Sum1/1

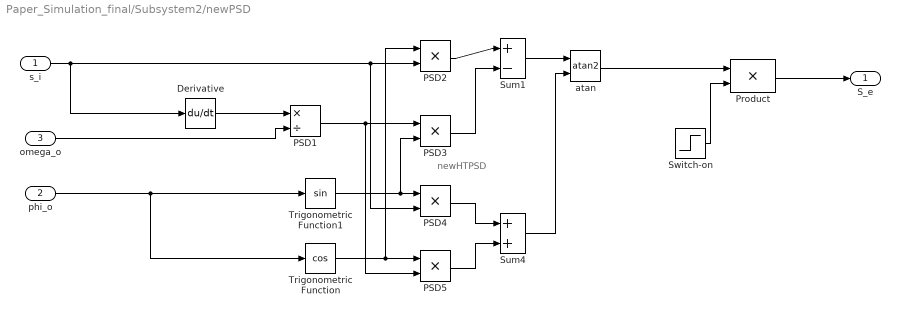
== system Paper_Simulation_final/Subsystem2/newPSD ==
  note: newHTPSD
  s_i : Inport
  phi_o : Inport  Port=2
  omega_o : Inport  Port=3
  Derivative : Derivative
  PSD1 : Product  Inputs=*/  InputSameDT=on  SaturateOnIntegerOverflow=on  OutDataTypeStr=Inherit: Same as first input
  PSD{2..5} (4 alike) : Product  Inputs=**  InputSameDT=on  SaturateOnIntegerOverflow=on  OutDataTypeStr=Inherit: Same as first input
  Product : Product  InputSameDT=on  SaturateOnIntegerOverflow=on  OutDataTypeStr=Inherit: Same as first input
  Sum1 : Sum  Inputs=|+-  InputSameDT=on  SaturateOnIntegerOverflow=on  OutDataTypeStr=Inherit: Same as first input
  Sum4 : Sum  InputSameDT=on  SaturateOnIntegerOverflow=on  OutDataTypeStr=Inherit: Same as first input
  Switch-on : Step  Time=Tsw+tstop  SampleTime=0
  Trigonometric Function : Trigonometry  Operator=cos
  Trigonometric Function1 : Trigonometry
  atan : Trigonometry  Operator=atan2
  S_e : Outport
  wires:
  omega_o/1 -> PSD1/2
  PSD1/1 -> PSD5/2, PSD3/1
  Derivative/1 -> PSD1/1
  PSD2/1 -> Sum1/1
  PSD3/1 -> Sum1/2
  Sum1/1 -> atan/1
  PSD4/1 -> Sum4/1
  PSD5/1 -> Sum4/2
  Sum4/1 -> atan/2
  s_i/1 -> PSD4/2, PSD2/2, Derivative/1
  Trigonometric Function/1 -> PSD2/1, PSD5/1
  Trigonometric Function1/1 -> PSD3/2, PSD4/1
  phi_o/1 -> Trigonometric Function1/1, Trigonometric Function/1
  atan/1 -> Product/1
  Product/1 -> S_e/1
  Switch-on/1 -> Product/2

== system Paper_Simulation_final/Design/Subsystem/Subsystem ==
  Plant Gain : Inport
  Constant : Constant  Value=a
  Constant1 : Constant
  Divide : Product  Inputs=/
  Product : Product
  Sqrt : Sqrt  SaturateOnIntegerOverflow=on
  Square : Math  Operator=square  SaturateOnIntegerOverflow=on
  Sum : Sum  Inputs=|++
  K : Outport
  wires:
  Divide/1 -> K/1
  Sum/1 -> Sqrt/1
  Square/1 -> Sum/1
  Sqrt/1 -> Product/1
  Plant Gain/1 -> Product/2
  Constant/1 -> Square/1
  Product/1 -> Divide/1
  Constant1/1 -> Sum/2

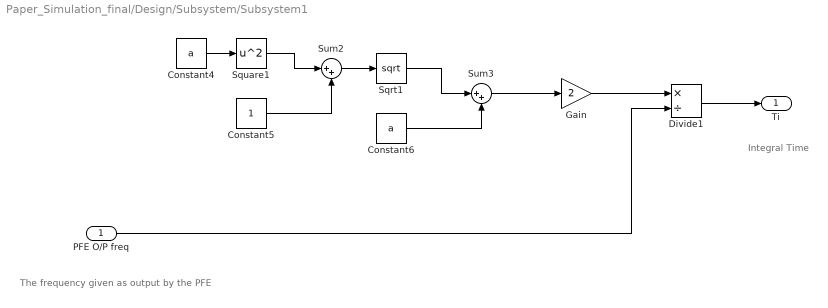
== system Paper_Simulation_final/Design/Subsystem/Subsystem1 ==
  note: Integral Time
  note: The frequency given as output by the PFE
  PFE O/P freq : Inport
  Constant4 : Constant  Value=a
  Constant5 : Constant
  Constant6 : Constant  Value=a
  Divide1 : Product  Inputs=*/
  Gain : Gain  Gain=2
  Sqrt1 : Sqrt  SaturateOnIntegerOverflow=on
  Square1 : Math  Operator=square  SaturateOnIntegerOverflow=on
  Sum2 : Sum  Inputs=|++
  Sum3 : Sum  Inputs=|++
  Ti : Outport
  wires:
  Constant6/1 -> Sum3/2
  PFE O/P freq/1 -> Divide1/2
  Sum3/1 -> Gain/1
  Gain/1 -> Divide1/1
  Sum2/1 -> Sqrt1/1
  Constant5/1 -> Sum2/2
  Constant4/1 -> Square1/1
  Sqrt1/1 -> Sum3/1
  Square1/1 -> Sum2/1
  Divide1/1 -> Ti/1

== system Paper_Simulation_final/GE/Amplitude Estimator/Hilbert Filter ==
  In : Inport
  Generated Filter Block : DiscreteFir  Tag=BlockMethodSubSystem  Coefficients=[-0.026449858259791379 -0.00578355491829027 -0.016572261903348456 -0.0095390561131982743 -0.022461390535071568 -0.014999256435125952 -0.030323967074738556 -0.023012528163449009 -0.041429315821655127 -0.035762828939278346 -0.05911752381753177 -0.059034685410808696 -0.094459906652176406 -0.11739830204172252 -0.21797718993610349 -0.62869353747279177 0.62869353747279177 0.21797718993610349 0.11739830204172252 0.094459906652176406 0.059034685410808696 0.05911752381753177 0.035762828939278346 0.041429315821655127 0.023012528163449009 0.030323967074738556 0.014999256435125952 0.022461390535071568 0.0095390561131982743 0.016572261903348456 0.00578355491829027 0.026449858259791379]  InputProcessing=Columns as channels (frame based)
  Out : Outport  VectorParamsAs1DForOutWhenUnconnected=off
  wires:
  Generated Filter Block/1 -> Out/1
  In/1 -> Generated Filter Block/1

== system Paper_Simulation_final/GE/Amplitude Estimator/Subsystem ==
  x : Inport
  omega_1 : Inport  Port=2
  VBPF : Subsystem
  y : Outport
  wires:
  omega_1/1 -> VBPF/2(W1)
  x/1 -> VBPF/1(X)
  VBPF/1(y) -> y/1

== system Paper_Simulation_final/GE/Amplitude Estimator _ for plant output/Hilbert Filter ==
  In : Inport
  Generated Filter Block : DiscreteFir  Tag=BlockMethodSubSystem  Coefficients=[-0.026449858259791379 -0.00578355491829027 -0.016572261903348456 -0.0095390561131982743 -0.022461390535071568 -0.014999256435125952 -0.030323967074738556 -0.023012528163449009 -0.041429315821655127 -0.035762828939278346 -0.05911752381753177 -0.059034685410808696 -0.094459906652176406 -0.11739830204172252 -0.21797718993610349 -0.62869353747279177 0.62869353747279177 0.21797718993610349 0.11739830204172252 0.094459906652176406 0.059034685410808696 0.05911752381753177 0.035762828939278346 0.041429315821655127 0.023012528163449009 0.030323967074738556 0.014999256435125952 0.022461390535071568 0.0095390561131982743 0.016572261903348456 0.00578355491829027 0.026449858259791379]  InputProcessing=Columns as channels (frame based)
  Out : Outport  VectorParamsAs1DForOutWhenUnconnected=off
  wires:
  Generated Filter Block/1 -> Out/1
  In/1 -> Generated Filter Block/1

== system Paper_Simulation_final/GE/Amplitude Estimator _ for plant output/Subsystem ==
  x : Inport
  omega_o : Inport  Port=2
  VBPF : Subsystem
  y : Outport
  wires:
  omega_o/1 -> VBPF/2(wo)
  x/1 -> VBPF/1(X)
  VBPF/1(y) -> y/1

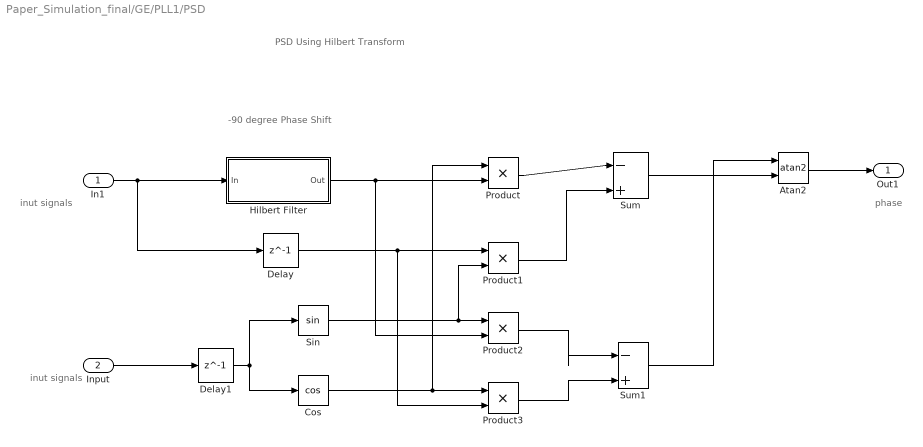
== system Paper_Simulation_final/GE/PLL1/PSD ==
  note: inut signals
  note: phase
  note: -90 degree Phase Shift
  note: PSD Using Hilbert Transform
  note: inut signals
  In1 : Inport
  Input : Inport  Port=2
  Atan2 : Trigonometry  Operator=atan2
  Cos : Trigonometry  Operator=cos
  Delay : Delay  DelayLength=1
  Delay1 : Delay  DelayLength=1
  Hilbert Filter : Subsystem  DialogController=fdesignblkfcn  InitFcn=fdesignblkfcn(gcbh, {'InitFcn'});  mask(Hilbert Filter){}
      mask help: Design a Hilbert filter
      settings: CopyFcn=fdesignblkfcn(gcbh, {'CopyFcn'});
      mask Help: helpview(mapfilelocation('dsp'), 'dsphilbertfilter');
      mask Display: disp('Hilbert')
  Product{,1..3} (4 alike) : Product
  Sin : Trigonometry
  Sum : Sum  Inputs=|-+
  Sum1 : Sum  Inputs=|-+
  Out1 : Outport
  wires:
  In1/1 -> Delay/1, Hilbert Filter/1(In)
  Hilbert Filter/1(Out) -> Product2/2, Product/2
  Input/1 -> Delay1/1
  Delay1/1 -> Sin/1, Cos/1
  Sin/1 -> Product1/2, Product2/1
  Cos/1 -> Product/1, Product3/1
  Delay/1 -> Product3/2, Product1/1
  Product/1 -> Sum/1
  Product1/1 -> Sum/2
  Atan2/1 -> Out1/1
  Sum/1 -> Atan2/2
  Product2/1 -> Sum1/1
  Product3/1 -> Sum1/2
  Sum1/1 -> Atan2/1

== system Paper_Simulation_final/Subsystem2/AMPu/VBPF ==
  x : Inport
  omega_0 : Inport  Port=2
  Integrator : Integrator
  Integrator1 : Integrator
  Product : Product  InputSameDT=on  SaturateOnIntegerOverflow=on  OutDataTypeStr=Inherit: Same as first input
  Product1 : Product  InputSameDT=on  SaturateOnIntegerOverflow=on  OutDataTypeStr=Inherit: Same as first input
  Sum : Sum  Inputs=|-+  InputSameDT=on  SaturateOnIntegerOverflow=on  OutDataTypeStr=Inherit: Same as first input
  Sum1 : Sum  Inputs=|+-  InputSameDT=on  SaturateOnIntegerOverflow=on  OutDataTypeStr=Inherit: Same as first input
  beta : Gain  Gain=0.1*beta  SaturateOnIntegerOverflow=on  OutDataTypeStr=Inherit: Same as input  ParamDataTypeStr=Inherit: Same as input
  y : Outport
  wires:
  beta/1 -> Sum/2
  Sum1/1 -> beta/1
  Product/1 -> Integrator/1
  Integrator1/1 -> Sum/1
  Product1/1 -> Integrator1/1
  Integrator/1 -> Sum1/2, y/1, Product1/1
  omega_0/1 -> Product/2, Product1/2
  Sum/1 -> Product/1
  x/1 -> Sum1/1

== system Paper_Simulation_final/Subsystem2/AMPy/VBPF ==
  x : Inport
  omega_0 : Inport  Port=2
  Integrator : Integrator
  Integrator1 : Integrator
  Product : Product  InputSameDT=on  SaturateOnIntegerOverflow=on  OutDataTypeStr=Inherit: Same as first input
  Product1 : Product  InputSameDT=on  SaturateOnIntegerOverflow=on  OutDataTypeStr=Inherit: Same as first input
  Sum : Sum  Inputs=|-+  InputSameDT=on  SaturateOnIntegerOverflow=on  OutDataTypeStr=Inherit: Same as first input
  Sum1 : Sum  Inputs=|+-  InputSameDT=on  SaturateOnIntegerOverflow=on  OutDataTypeStr=Inherit: Same as first input
  beta : Gain  Gain=0.1*beta  SaturateOnIntegerOverflow=on  OutDataTypeStr=Inherit: Same as input  ParamDataTypeStr=Inherit: Same as input
  y : Outport
  wires:
  x/1 -> Sum1/1
  Sum/1 -> Product/1
  omega_0/1 -> Product1/2, Product/2
  Integrator/1 -> Product1/1, y/1, Sum1/2
  Product1/1 -> Integrator1/1
  Integrator1/1 -> Sum/1
  Product/1 -> Integrator/1
  Sum1/1 -> beta/1
  beta/1 -> Sum/2

== system Paper_Simulation_final/GE/Amplitude Estimator/Subsystem/VBPF ==
  note: W1 from PFE
  note: USES OF VBPF
  note: (i) elimination of DC Values
      | (ii) attenuation of harmonics, arising for example if there
      | are nonlinearities in the plant or actuator
      | (iii) reduction in the effect of additive noise.
  note: VBPF
  X : Inport
  W1 : Inport  Port=2
  Beta : Gain  Gain=0.15
  Integrator : Integrator
  Integrator1 : Integrator  LimitOutput=on  UpperSaturationLimit=1000  LowerSaturationLimit=-1000  AbsoluteTolerance=1000
  Product : Product
  Product1 : Product
  Sum : Sum  Inputs=|+-
  Sum1 : Sum  Inputs=|-+
  y : Outport
  wires:
  X/1 -> Sum/1
  Sum/1 -> Beta/1
  Integrator/1 -> Sum1/1
  Beta/1 -> Sum1/2
  Sum1/1 -> Product/1
  W1/1 -> Product1/2, Product/2
  Product/1 -> Integrator1/1
  Product1/1 -> Integrator/1
  Integrator1/1 -> Product1/1, Sum/2, y/1

== system Paper_Simulation_final/GE/Amplitude Estimator _ for plant output/Subsystem/VBPF ==
  note: USES OF VBPF
  note: (i) elimination of DC Values
      | (ii) attenuation of harmonics, arising for example if there
      | are nonlinearities in the plant or actuator
      | (iii) reduction in the effect of additive noise.
  note: VBPF
  X : Inport
  wo : Inport  Port=2
  Beta : Gain  Gain=0.15
  Integrator : Integrator
  Integrator1 : Integrator
  Product : Product
  Product1 : Product
  Sum : Sum  Inputs=|+-
  Sum1 : Sum  Inputs=|-+
  y : Outport
  wires:
  X/1 -> Sum/1
  Sum/1 -> Beta/1
  Integrator/1 -> Sum1/1
  Beta/1 -> Sum1/2
  Sum1/1 -> Product/1
  wo/1 -> Product1/2, Product/2
  Product/1 -> Integrator1/1
  Integrator1/1 -> Product1/1, Sum/2, y/1
  Product1/1 -> Integrator/1

== system Paper_Simulation_final/GE/PLL1/PSD/Hilbert Filter ==
  In : Inport
  Generated Filter Block : DiscreteFir  Tag=BlockMethodSubSystem  Coefficients=[-0.026449858259791379 -0.00578355491829027 -0.016572261903348456 -0.0095390561131982743 -0.022461390535071568 -0.014999256435125952 -0.030323967074738556 -0.023012528163449009 -0.041429315821655127 -0.035762828939278346 -0.05911752381753177 -0.059034685410808696 -0.094459906652176406 -0.11739830204172252 -0.21797718993610349 -0.62869353747279177 0.62869353747279177 0.21797718993610349 0.11739830204172252 0.094459906652176406 0.059034685410808696 0.05911752381753177 0.035762828939278346 0.041429315821655127 0.023012528163449009 0.030323967074738556 0.014999256435125952 0.022461390535071568 0.0095390561131982743 0.016572261903348456 0.00578355491829027 0.026449858259791379]  InputProcessing=Columns as channels (frame based)
  Out : Outport  VectorParamsAs1DForOutWhenUnconnected=off
  wires:
  Generated Filter Block/1 -> Out/1
  In/1 -> Generated Filter Block/1
